simulink model "TractionSystem"  (R2019b)
settings: configuration reference "ConfigSet_TractionSystem_Reference" (kept outside this file)
model workspace (MAT data in the model file):
  Prm_TractionSystem = Simulink.Parameter
  Prm_TractionSystem.Value.DesignMaxTractionTorque = 1091
  Prm_TractionSystem.Value.DesignMaxTractionPower = 210120
  Prm_TractionSystem.Value.DesignTimeToMaxTraction = 1.75
  Prm_TractionSystem.Value.DesignMaxBrakingTorque = 1570
  Prm_TractionSystem.Value.DesignMaxBrakingPower = 430000
  Prm_TractionSystem.Value.BrakeFadeRampDownSpeeds = [0.3 1]
  Prm_TractionSystem.Value.DesignGearingRatio = 6.79
  Prm_TractionSystem.Value.DesignGearingEfficiency = 0.97
  Prm_TractionSystem.Value.DesignWheelDiameter = 0.82
  Prm_TractionSystem.Value.DesignBogieMotorCount = 2
  Prm_TractionSystem.Value.AxleHasMotor = [1 1]
  Prm_TractionSystem.Value.EmergencyBrakeDeactivatesDynamicBrake = 1
  Prm_TractionSystem.Value.WheelSlipProtectionEnable = 1
  Prm_TractionSystem.Value.WheelSlideProtectionEnable = 1
  Prm_TractionSystem.Value.JerkLimit = 0.75
  Prm_TractionSystem.Value.MaxContinuousSlipBeforeTractionCutout = 10
  Prm_TractionSystem.Value.MaxContinuousSlideBeforeBrakeCutout = 10
  Prm_TractionSystem.DataType = 'Bus: BD_TractionSystem_Prm'
  Prm_TractionSystem.Dimensions = [1 1]
  SampleTime = 0.01
undefined symbols (not defined in the file): Audio, BCU, Bogie, BogieNotIsolated, DiscIntNeverNeededParam, Dynamics, EDBrakeStatus, EDBrakingEffortAchieved, EDBrakingEffortPossible, ElectricalSystem, Forward, MaxAxles, Reverse, TCMS, TCUWheelSlideControlActive, TractionContactorStatus, TractionControl, TractionEDPower, Trafo_TCU, VehicleBogieDerailed, VehicleDerailed, WheelAngularVelocity
libraries: simulink x19, LatchesLib x3, TimersLib x2, WheelSlipControl_Lib x2, simulink_extras x2, TractionLib x2
(part 1 of 2)
settings Model: ParameterArgumentNames=Prm_TractionSystem  Creator=cdyer  LastModifiedBy=hinganes
settings ConfigSetRef: SourceName=ConfigSet_TractionSystem_Reference  SourceLocation=Base Workspace

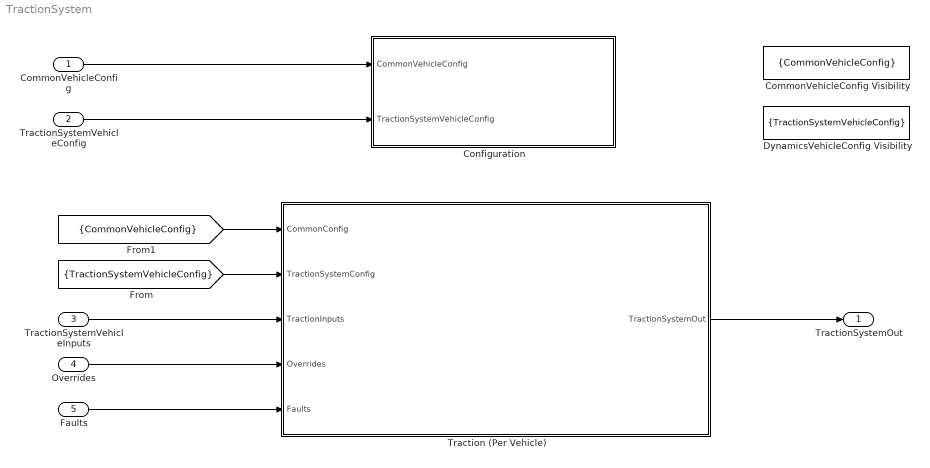
== system TractionSystem ==
  CommonVehicleConfig : Inport  OutDataTypeStr=Bus: BD_CommonTrain_Cfg_Vehicle  PortDimensions=MaxVehicles  BusOutputAsStruct=on
  TractionSystemVehicleConfig : Inport  Port=2  OutDataTypeStr=Bus: BD_TractionSystem_Cfg_Vehicle  BusOutputAsStruct=on
  TractionSystemVehicleInputs : Inport  Port=3  OutDataTypeStr=Bus: BD_TractionSystem_In_Vehicle  BusOutputAsStruct=on
  Overrides : Inport  Port=4  OutDataTypeStr=Bus: BD_TractionSystem_In_Overrides  BusOutputAsStruct=on
  Faults : Inport  Port=5  OutDataTypeStr=Bus: BD_TractionSystem_In_Faults  BusOutputAsStruct=on
  CommonVehicleConfig Visibility : GotoTagVisibility  GotoTag=CommonVehicleConfig
  Configuration : Subsystem
  DynamicsVehicleConfig Visibility : GotoTagVisibility  GotoTag=TractionSystemVehicleConfig
  Traction (Per Vehicle) : Subsystem  TreatAsAtomicUnit=on
  TractionSystemOut : Outport  OutDataTypeStr=Bus: BD_TractionSystem_Out_Vehicle  VectorParamsAs1DForOutWhenUnconnected=off  BusOutputAsStruct=on
  wires:
  Traction (Per Vehicle)/1(TractionSystemOut) -> TractionSystemOut/1
  CommonVehicleConfig/1 -> Configuration/1(CommonVehicleConfig)
  TractionSystemVehicleInputs/1 -> Traction (Per Vehicle)/3(TractionInputs)
  TractionSystemVehicleConfig/1 -> Configuration/2(TractionSystemVehicleConfig)
  [CommonVehicleConfig] -> Traction (Per Vehicle)/1(CommonConfig)
  [TractionSystemVehicleConfig] -> Traction (Per Vehicle)/2(TractionSystemConfig)
  Overrides/1 -> Traction (Per Vehicle)/4(Overrides)
  Faults/1 -> Traction (Per Vehicle)/5(Faults)

== system TractionSystem/Configuration ==
  CommonVehicleConfig : Inport  OutDataTypeStr=Bus: BD_CommonTrain_Cfg_Vehicle  BusOutputAsStruct=on
  TractionSystemVehicleConfig : Inport  Port=2  OutDataTypeStr=Bus: BD_TractionSystem_Cfg_Vehicle  BusOutputAsStruct=on
  ConfigProcessing : Subsystem
  Step : Step  Before=1  After=0  SampleTime=SampleTime
  tag scope: CommonVehicleConfig=scoped, TractionSystemVehicleConfig=scoped
  wires:
  Step/1 -> ConfigProcessing/Enable
  CommonVehicleConfig/1 -> ConfigProcessing/1(In1)
  TractionSystemVehicleConfig/1 -> ConfigProcessing/2(In2)
  ConfigProcessing/1(CommonVehicleConfig) -> [CommonVehicleConfig]
  ConfigProcessing/2(TractionSystemVehicleConfig) -> [TractionSystemVehicleConfig]

== system TractionSystem/Traction (Per Vehicle) ==
  CommonConfig : Inport  Partition=on  PartitionDimension=1  PartitionWidth=1  PartitionOffset=0
  TractionSystemConfig : Inport  Port=2  Partition=on  PartitionDimension=1  PartitionWidth=1  PartitionOffset=0
  TractionInputs : Inport  Port=3  Partition=on  PartitionDimension=1  PartitionWidth=1  PartitionOffset=0
  Overrides : Inport  Port=4  Partition=on  PartitionDimension=1  PartitionWidth=1  PartitionOffset=0
  Faults : Inport  Port=5  Partition=on  PartitionDimension=1  PartitionWidth=1  PartitionOffset=0
  AND : Logic  AllPortsSameDT=off  OutDataTypeStr=boolean
  Bus Selector : BusSelector  OutputSignals=HasMotors
  Bus Selector1 : BusSelector  OutputSignals=Enabled
  ForEachVehicle : ForEach  DisableCoverage=on
  MotorVehicle : Subsystem
  TractionSystemOut : Outport  ConcatenationDimension=1  VectorParamsAs1DForOutWhenUnconnected=off
  wires:
  TractionSystemConfig/1 -> Bus Selector/1
  TractionInputs/1 -> MotorVehicle/2(TractionInputs)
  MotorVehicle/1(TractionSystemOut) -> TractionSystemOut/1
  CommonConfig/1 -> Bus Selector1/1, MotorVehicle/1(CommonConfig)
  Overrides/1 -> MotorVehicle/3(Overrides)
  Faults/1 -> MotorVehicle/4(Faults)
  Bus Selector/1 -> AND/1  "<HasMotors>"
  Bus Selector1/1 -> AND/2  "<Enabled>"
  AND/1 -> MotorVehicle/Enable

== system TractionSystem/Configuration/ConfigProcessing ==
  In1 : Inport
  In2 : Inport  Port=2
  Enable : EnablePort
  ConfigCheck : Subsystem
  CommonVehicleConfig : Outport  VectorParamsAs1DForOutWhenUnconnected=off  BusOutputAsStruct=on
  TractionSystemVehicleConfig : Outport  Port=2  VectorParamsAs1DForOutWhenUnconnected=off  BusOutputAsStruct=on
  wires:
  In1/1 -> ConfigCheck/1(In1)
  In2/1 -> ConfigCheck/2(In2)
  ConfigCheck/1(CommonVehicleConfig) -> CommonVehicleConfig/1
  ConfigCheck/2(TractionSystemVehicleConfig) -> TractionSystemVehicleConfig/1

== system TractionSystem/Traction (Per Vehicle)/MotorVehicle ==
  CommonConfig : Inport
  TractionInputs : Inport  Port=2
  Overrides : Inport  Port=3
  Faults : Inport  Port=4
  MotorVehicleEnable : EnablePort
  OutputAdapter : Subsystem
  Unit Delay : UnitDelay  SampleTime=-1  HasFrameUpgradeWarning=on
  VehicleTractionControlUnit : Subsystem
  VehicleTractionConvertersSystem : Subsystem
  TractionSystemOut : Outport  VectorParamsAs1DForOutWhenUnconnected=off
  wires:
  Faults/1 -> VehicleTractionConvertersSystem/5(Faults), VehicleTractionControlUnit/2(Faults)
  Overrides/1 -> VehicleTractionControlUnit/3(Overrides), VehicleTractionConvertersSystem/4(Overrides)
  CommonConfig/1 -> VehicleTractionConvertersSystem/3(CommonConfig)
  VehicleTractionControlUnit/2(TractionConverterControl) -> VehicleTractionConvertersSystem/1(TractionConverterControlIn)
  VehicleTractionConvertersSystem/2(BogieOutputs) -> Unit Delay/1
  Unit Delay/1 -> VehicleTractionControlUnit/4(TractionConvertersFB)
  VehicleTractionConvertersSystem/1(VehicleTractiveBrakingEffortPerAxle) -> OutputAdapter/3(VehicleTractiveBrakingEffortPerAxle)
  OutputAdapter/1(TractionSystemOut) -> TractionSystemOut/1
  TractionInputs/1 -> VehicleTractionConvertersSystem/2(TractionInputs), VehicleTractionControlUnit/1(TractionInputs), OutputAdapter/1(TractionInputs)
  VehicleTractionControlUnit/1(TractionControlUnitOut) -> OutputAdapter/2(TractionControlUnitOut)

== system TractionSystem/Configuration/ConfigProcessing/ConfigCheck ==
  In1 : Inport  Partition=on  PartitionDimension=1  PartitionWidth=1  PartitionOffset=0
  In2 : Inport  Port=2  Partition=on  PartitionDimension=1  PartitionWidth=1  PartitionOffset=0
  Bus Creator1 : BusCreator  Inputs=1  OutDataTypeStr=Bus: BD_TractionSystem_Cfg_Vehicle  NonVirtualBus=on
      settings: InheritFromInputs=off
  Bus Creator2 : BusCreator  Inputs=15  OutDataTypeStr=Bus: BD_CommonTrain_Cfg_Vehicle  NonVirtualBus=on
      settings: InheritFromInputs=off
  Bus Selector1 : BusSelector  OutputSignals=HasMotors
  Bus Selector3 : BusSelector  OutputSignals=Enabled,VehicleID,Type,Class,Orientation,Length,Height,Width,TareMass,GrossMass,LoadingMass,NumberOfAxles,NumberOfDrivenAxles,NumberOfBrakedAxles,WheelDiameter
  Data Type Conversion : DataTypeConversion
  Default Gearing Ratio : Subsystem
  Default Gross1 : Subsystem
  Default Height1 : Subsystem
  Default Length1 : Subsystem
  Default NumberOfAxles3 : Subsystem
  Default NumberOfAxles4 : Subsystem
  Default NumberOfAxles5 : Subsystem
  Default Tare1 : Subsystem
  Default WheelDiameter : Subsystem
  Default Width1 : Subsystem
  For Each : ForEach  DisableCoverage=on
  CommonVehicleConfig : Outport  ConcatenationDimension=1  VectorParamsAs1DForOutWhenUnconnected=off
  TractionSystemVehicleConfig : Outport  Port=2  ConcatenationDimension=1  VectorParamsAs1DForOutWhenUnconnected=off
  wires:
  In2/1 -> Bus Selector1/1
  Bus Selector1/1 -> Default Gearing Ratio/1(In1)  "<HasMotors>"
  Data Type Conversion/1 -> Bus Creator1/1  "HasMotors"
  Bus Creator1/1 -> TractionSystemVehicleConfig/1
  In1/1 -> Bus Selector3/1
  Bus Selector3/3 -> Bus Creator2/3  "<Type>"
  Bus Selector3/4 -> Bus Creator2/4  "<Class>"
  Bus Selector3/5 -> Bus Creator2/5  "<Orientation>"
  Bus Selector3/6 -> Default Length1/1(In1)  "<Length>"
  Bus Selector3/7 -> Default Height1/1(In1)  "<Height>"
  Bus Selector3/8 -> Default Width1/1(In1)  "<Width>"
  Bus Selector3/9 -> Default Tare1/1(In1)  "<TareMass>"
  Bus Selector3/10 -> Default Gross1/1(In1)  "<GrossMass>"
  Bus Selector3/11 -> Bus Creator2/11  "<LoadingMass>"
  Default Length1/1(Out1) -> Bus Creator2/6  "Length"
  Bus Creator2/1 -> CommonVehicleConfig/1
  Default Height1/1(Out1) -> Bus Creator2/7  "Height"
  Default Width1/1(Out1) -> Bus Creator2/8  "Width"
  Default Tare1/1(Out1) -> Bus Creator2/9  "TareMass"
  Default Gross1/1(Out1) -> Bus Creator2/10  "GrossMass"
  Bus Selector3/12 -> Default NumberOfAxles3/1(In)  "<NumberOfAxles>"
  Default NumberOfAxles3/1(Out) -> Bus Creator2/12  "NumberOfAxles"
  Bus Selector3/13 -> Default NumberOfAxles4/1(In)  "<NumberOfDrivenAxles>"
  Bus Selector3/14 -> Default NumberOfAxles5/1(In)  "<NumberOfBrakedAxles>"
  Default NumberOfAxles5/1(Out) -> Bus Creator2/14  "NumberOfBrakedAxles"
  Default NumberOfAxles4/1(Out) -> Bus Creator2/13  "NumberOfDrivenAxles"
  Bus Selector3/15 -> Default WheelDiameter/1(In)  "<WheelDiameter>"
  Bus Selector3/1 -> Bus Creator2/1  "<Enabled>"
  Default WheelDiameter/1(Out) -> Bus Creator2/15  "WheelDiameter"
  Bus Selector3/2 -> Bus Creator2/2  "<VehicleID>"
  Default Gearing Ratio/1(Out1) -> Data Type Conversion/1  "HasMotors"

== system TractionSystem/Traction (Per Vehicle)/MotorVehicle/OutputAdapter ==
  TractionInputs : Inport
  TractionControlUnitOut : Inport  Port=2
  VehicleTractiveBrakingEffortPerAxle : Inport  Port=3
  AudioOutputsRepack : Subsystem
  Bus Assignment : BusAssignment  AssignedSignals=TractionControl,Dynamics,Audio
  Constant1 : Constant  Value=0  OutDataTypeStr=Bus: BD_TractionSystem_Out_Vehicle
  DynamicsOutputsRepack : Subsystem
  TractionSystemOut : Outport  VectorParamsAs1DForOutWhenUnconnected=off
  wires:
  Bus Assignment/1 -> TractionSystemOut/1
  Constant1/1 -> Bus Assignment/1
  VehicleTractiveBrakingEffortPerAxle/1 -> AudioOutputsRepack/1(In1), DynamicsOutputsRepack/1(VehicleTractiveBrakingEffortPerAxle)
  DynamicsOutputsRepack/1(DynamicsTractionBrakingForce) -> Bus Assignment/3
  TractionInputs/1 -> AudioOutputsRepack/2(TractionInputs)
  AudioOutputsRepack/1(Out1) -> Bus Assignment/4
  TractionControlUnitOut/1 -> Bus Assignment/2

== system TractionSystem/Traction (Per Vehicle)/MotorVehicle/VehicleTractionControlUnit ==
  TractionInputs : Inport
  Faults : Inport  Port=2
  Overrides : Inport  Port=3
  TractionConvertersFB : Inport  Port=4
  Bus Selector : BusSelector  OutputSignals=ElectricalSystem,Dynamics,TCMS
  Bus Selector1 : BusSelector  OutputSignals=ForwardTW,ReverseTW,TractionActiveTW,NoEmergencyBrakeActiveTW,VCBState,ContactorsFailure,Bogie
  Bus Selector2 : BusSelector  OutputSignals=Velocity,Bogie
  Bus Selector3 : BusSelector  OutputSignals=TCMSTractionCmd,TCMSEDBrakingCmd,Bogie
  Bus Selector4 : BusSelector  OutputSignals=Bogie
  OutputAdapter : Subsystem
  Subsystem : Subsystem
  Sum of Elements : Sum  Inputs=+
  Terminator : Terminator
  TractionControl (Per Bogie) : Subsystem
  TractionConverterCircuits : Subsystem
  TractionControlUnitOut : Outport  VectorParamsAs1DForOutWhenUnconnected=off
  TractionConverterControl : Outport  Port=2  VectorParamsAs1DForOutWhenUnconnected=off
  wires:
  TractionInputs/1 -> Bus Selector/1
  Faults/1 -> TractionControl (Per Bogie)/15(Faults), OutputAdapter/6(Faults), Bus Selector4/1, TractionConverterCircuits/3(Faults)
  Overrides/1 -> TractionControl (Per Bogie)/13(Overrides)
  TractionConvertersFB/1 -> Subsystem/1(In1), TractionControl (Per Bogie)/14(TractionConvertersFB)
  TractionControl (Per Bogie)/2(TCUtoElectricalOutputs) -> OutputAdapter/1(TCUtoElectricalOut)
  TractionControl (Per Bogie)/1(TractionConverterControl) -> TractionConverterControl/1
  Bus Selector/1 -> Bus Selector1/1  "<ElectricalSystem>"
  Bus Selector/2 -> Bus Selector2/1  "<Dynamics>"
  Bus Selector/3 -> Bus Selector3/1  "<TCMS>"
  Bus Selector1/1 -> TractionControl (Per Bogie)/1(ForwardTW)  "<ForwardTW>"
  Bus Selector1/2 -> TractionControl (Per Bogie)/2(ReverseTW)  "<ReverseTW>"
  Bus Selector1/3 -> TractionControl (Per Bogie)/3(TractionActive)  "<TractionActiveTW>"
  Bus Selector1/4 -> TractionControl (Per Bogie)/4(NoEmergencyBrakeActive)  "<NoEmergencyBrakeActiveTW>"
  Bus Selector1/7 -> TractionControl (Per Bogie)/6(BogieElectrical)  "<Bogie>"
  Bus Selector2/1 -> TractionControl (Per Bogie)/7(Velocity)  "<Velocity>"
  Bus Selector2/2 -> TractionControl (Per Bogie)/8(BogieDynamics)  "<Bogie>"
  Bus Selector3/1 -> TractionControl (Per Bogie)/9(TCMSTractionCmd)  "<TCMSTractionCmd>"
  Bus Selector3/2 -> TractionControl (Per Bogie)/10(TCMSEDBrakingCmd)  "<TCMSEDBrakingCmd>"
  TractionControl (Per Bogie)/4(TCUToBCUOutputs) -> OutputAdapter/3(TCUtoBCUOut)
  Bus Selector3/3 -> TractionControl (Per Bogie)/11(TCMSBogie)  "<Bogie>"
  TractionControl (Per Bogie)/3(TCUtoTCMSOutputs) -> OutputAdapter/2(TCUtoTCMSOut)
  OutputAdapter/1(TractionControlUnitOut) -> TractionControlUnitOut/1
  Bus Selector4/1 -> TractionControl (Per Bogie)/12(BogieFaults)  "<Bogie>"
  Bus Selector1/5 -> TractionConverterCircuits/1(VCB State)  "<VCBState>"
  TractionConverterCircuits/1(TMPower) -> [ContactorStatus], TractionControl (Per Bogie)/5(TMPower)
  TractionConverterCircuits/2(Trafo_TCU) -> OutputAdapter/5(Trafo_TCU)
  Sum of Elements/1 -> Terminator/1  "VehicleTractivePower"
  Subsystem/1(<BogieTractivePower>) -> Sum of Elements/1
  Bus Selector1/6 -> TractionConverterCircuits/2(ContactorFault)  "<ContactorsFailure>"
  [ContactorStatus] -> OutputAdapter/4(ContactorStatus)

== system TractionSystem/Traction (Per Vehicle)/MotorVehicle/VehicleTractionConvertersSystem ==
  TractionConverterControlIn : Inport
  Bus Element In : Inport  Port=2  PortName=TractionInputs  Element=Dynamics
  In Bus Element : Inport  Port=2  PortName=TractionInputs  Element=ElectricalSystem
  In Bus Element1 : Inport  Port=2  PortName=TractionInputs  Element=TCMS
  CommonConfig : Inport  Port=3
  Overrides : Inport  Port=4
  Faults : Inport  Port=5
  BogieTractionConverterSystem (Per Bogie) : Subsystem
  Bus Selector1 : BusSelector  OutputSignals=Bogie
  Bus Selector2 : BusSelector  OutputSignals=Orientation
  Bus Selector5 : BusSelector  OutputSignals=TractionForceVariation,DynamicBrakeForceVariation
  Terminator1 : Terminator
  VehicleTractiveBrakingEffortPerAxle : Outport  VectorParamsAs1DForOutWhenUnconnected=off
  BogieOutputs : Outport  Port=2  VectorParamsAs1DForOutWhenUnconnected=off
  wires:
  TractionConverterControlIn/1 -> BogieTractionConverterSystem (Per Bogie)/1(BogieTractionConverterControlIn)
  Bus Element In/1 -> Bus Selector1/1
  Overrides/1 -> Bus Selector5/1
  CommonConfig/1 -> Bus Selector2/1
  Bus Selector5/1 -> BogieTractionConverterSystem (Per Bogie)/4(TractionEffortVariationOverride)  "<TractionForceVariation>"
  Bus Selector5/2 -> BogieTractionConverterSystem (Per Bogie)/5(BrakingEffortVariationOverride)  "<DynamicBrakeForceVariation>"
  Bus Selector1/1 -> BogieTractionConverterSystem (Per Bogie)/3(BogieDynamics)  "<Bogie>"
  Bus Selector2/1 -> BogieTractionConverterSystem (Per Bogie)/6(Orientation)  "<Orientation>"
  BogieTractionConverterSystem (Per Bogie)/1(BogieForcesPerAxle) -> VehicleTractiveBrakingEffortPerAxle/1
  Faults/1 -> Terminator1/1
  BogieTractionConverterSystem (Per Bogie)/2(BogieOutputs) -> BogieOutputs/1
  In Bus Element/1 -> BogieTractionConverterSystem (Per Bogie)/2(MotorIn)
  In Bus Element1/1 -> BogieTractionConverterSystem (Per Bogie)/7(TCMS)

== system TractionSystem/Configuration/ConfigProcessing/ConfigCheck/Default Gearing Ratio ==
  In1 : Inport
  Default : Constant  Value=0
  Min Value : simulink/Logic and Bit Operations/Compare To Constant  relop=>  const=0  OutDataTypeStr=boolean
  Switch : Switch  Criteria=u2 > Threshold
  Out1 : Outport  VectorParamsAs1DForOutWhenUnconnected=off
  wires:
  In1/1 -> Min Value/1, Switch/1
  Min Value/1 -> Switch/2
  Default/1 -> Switch/3
  Switch/1 -> Out1/1

== system TractionSystem/Configuration/ConfigProcessing/ConfigCheck/Default Gross1 ==
  In1 : Inport
  Default : Constant  Value=16000
  Min Value : simulink/Logic and Bit Operations/Compare To Constant  relop=>  const=16000  OutDataTypeStr=boolean
  Switch : Switch  Criteria=u2 > Threshold
  Out1 : Outport  VectorParamsAs1DForOutWhenUnconnected=off
  wires:
  In1/1 -> Min Value/1, Switch/1
  Min Value/1 -> Switch/2
  Default/1 -> Switch/3
  Switch/1 -> Out1/1

== system TractionSystem/Configuration/ConfigProcessing/ConfigCheck/Default Height1 ==
  In1 : Inport
  Default : Constant  Value=3
  Min Value : simulink/Logic and Bit Operations/Compare To Constant  relop=>  const=0  OutDataTypeStr=boolean
  Switch : Switch  Criteria=u2 > Threshold
  Out1 : Outport  VectorParamsAs1DForOutWhenUnconnected=off
  wires:
  In1/1 -> Min Value/1, Switch/1
  Min Value/1 -> Switch/2
  Default/1 -> Switch/3
  Switch/1 -> Out1/1

== system TractionSystem/Configuration/ConfigProcessing/ConfigCheck/Default Length1 ==
  In1 : Inport
  Default : Constant  Value=20
  Min Value : simulink/Logic and Bit Operations/Compare To Constant  relop=>  const=0  OutDataTypeStr=boolean
  Switch : Switch  Criteria=u2 > Threshold
  Out1 : Outport  VectorParamsAs1DForOutWhenUnconnected=off
  wires:
  In1/1 -> Min Value/1, Switch/1
  Min Value/1 -> Switch/2
  Default/1 -> Switch/3
  Switch/1 -> Out1/1

== system TractionSystem/Configuration/ConfigProcessing/ConfigCheck/Default NumberOfAxles3 ==
  In : Inport
  Default : Constant  Value=6
  Min Value : simulink/Logic and Bit Operations/Compare To Constant  relop=>=  const=1  OutDataTypeStr=boolean
  Switch : Switch  Criteria=u2 > Threshold
  Out : Outport  VectorParamsAs1DForOutWhenUnconnected=off
  wires:
  Switch/1 -> Out/1
  Default/1 -> Switch/3
  Min Value/1 -> Switch/2
  In/1 -> Switch/1, Min Value/1

== system TractionSystem/Configuration/ConfigProcessing/ConfigCheck/Default NumberOfAxles4 ==
  In : Inport
  Default : Constant  Value=2
  Min Value : simulink/Logic and Bit Operations/Compare To Constant  relop=>=  const=1  OutDataTypeStr=boolean
  Switch : Switch  Criteria=u2 > Threshold
  Out : Outport  VectorParamsAs1DForOutWhenUnconnected=off
  wires:
  In/1 -> Min Value/1, Switch/1
  Min Value/1 -> Switch/2
  Default/1 -> Switch/3
  Switch/1 -> Out/1

== system TractionSystem/Configuration/ConfigProcessing/ConfigCheck/Default NumberOfAxles5 ==
  In : Inport
  Default : Constant  Value=2
  Min Value : simulink/Logic and Bit Operations/Compare To Constant  relop=>=  const=1  OutDataTypeStr=boolean
  Switch : Switch  Criteria=u2 > Threshold
  Out : Outport  VectorParamsAs1DForOutWhenUnconnected=off
  wires:
  Switch/1 -> Out/1
  Default/1 -> Switch/3
  Min Value/1 -> Switch/2
  In/1 -> Switch/1, Min Value/1

== system TractionSystem/Configuration/ConfigProcessing/ConfigCheck/Default Tare1 ==
  In1 : Inport
  Default : Constant  Value=16000
  Min Value : simulink/Logic and Bit Operations/Compare To Constant  relop=>  const=16000  OutDataTypeStr=boolean
  Switch : Switch  Criteria=u2 > Threshold
  Out1 : Outport  VectorParamsAs1DForOutWhenUnconnected=off
  wires:
  In1/1 -> Min Value/1, Switch/1
  Min Value/1 -> Switch/2
  Default/1 -> Switch/3
  Switch/1 -> Out1/1

== system TractionSystem/Configuration/ConfigProcessing/ConfigCheck/Default WheelDiameter ==
  In : Inport
  Default : Constant  Value=0.580
  Min Value : simulink/Logic and Bit Operations/Compare To Constant  relop=>  const=0  OutDataTypeStr=boolean
  Switch : Switch  Criteria=u2 > Threshold
  Out : Outport  VectorParamsAs1DForOutWhenUnconnected=off
  wires:
  In/1 -> Min Value/1, Switch/1
  Min Value/1 -> Switch/2
  Default/1 -> Switch/3
  Switch/1 -> Out/1

== system TractionSystem/Configuration/ConfigProcessing/ConfigCheck/Default Width1 ==
  In1 : Inport
  Default : Constant  Value=3
  Min Value : simulink/Logic and Bit Operations/Compare To Constant  relop=>  const=0  OutDataTypeStr=boolean
  Switch : Switch  Criteria=u2 > Threshold
  Out1 : Outport  VectorParamsAs1DForOutWhenUnconnected=off
  wires:
  In1/1 -> Min Value/1, Switch/1
  Min Value/1 -> Switch/2
  Default/1 -> Switch/3
  Switch/1 -> Out1/1

== system TractionSystem/Traction (Per Vehicle)/MotorVehicle/OutputAdapter/AudioOutputsRepack ==
  In1 : Inport
  TractionInputs : Inport  Port=2
  Bus Assignment1 : BusAssignment  AssignedSignals=TractionEDPower,WheelAngularVelocity
  Bus Selector : BusSelector  OutputSignals=Dynamics.Bogie
  Constant : Constant  Value=Prm_TractionSystem.DesignWheelDiameter
  Constant2 : Constant  Value=0  OutDataTypeStr=Bus: BD_TractionSystem_Out_Vehicle_Audio
  ForEachBogie : Subsystem  TreatAsAtomicUnit=on
  Gain : Gain  Gain=0.5
  IfWheelSlipping : MinMax  Function=max
  Product : Product  Inputs=*/
  Sum of Elements : Sum  Inputs=+
  Out1 : Outport
  wires:
  Gain/1 -> Product/2
  IfWheelSlipping/1 -> Product/1
  ForEachBogie/1(BogieTractionBrakingPower) -> Sum of Elements/1
  TractionInputs/1 -> Bus Selector/1
  ForEachBogie/2(BogieWheelSpeed) -> IfWheelSlipping/1
  Bus Selector/1 -> ForEachBogie/2(BogieDynamics)  "<Bogie>"
  Constant2/1 -> Bus Assignment1/1
  Product/1 -> Bus Assignment1/3  "WheelAngularSpeed"
  Sum of Elements/1 -> Bus Assignment1/2
  Constant/1 -> Gain/1
  Bus Assignment1/1 -> Out1/1
  In1/1 -> ForEachBogie/1(BogieTraction)

== system TractionSystem/Traction (Per Vehicle)/MotorVehicle/OutputAdapter/DynamicsOutputsRepack ==
  VehicleTractiveBrakingEffortPerAxle : Inport
  Assignment : Assignment  DiagnosticForDimensions=Warning  IndexOptions=Starting index (dialog)  Indices=1  OutputSizes=1
  Assignment1 : Assignment  DiagnosticForDimensions=Warning  IndexOptions=Starting index (dialog)  Indices=1  OutputSizes=1
  Assignment2 : Assignment  DiagnosticForDimensions=Warning  IndexOptions=Starting index (dialog)  Indices=1  OutputSizes=1
  Bus Creator : BusCreator  Inputs=3  OutDataTypeStr=Bus: BD_TractionSystem_Out_Vehicle_Dynamics  NonVirtualBus=on
  Constant : Constant  Value=zeros(1,MaxAxles)
  For Each Subsystem : Subsystem  TreatAsAtomicUnit=on
  DynamicsTractionBrakingForce : Outport
  wires:
  Constant/1 -> Assignment2/1, Assignment1/1, Assignment/1
  Bus Creator/1 -> DynamicsTractionBrakingForce/1
  Assignment/1 -> Bus Creator/1  "TractionBrakingForce"
  VehicleTractiveBrakingEffortPerAxle/1 -> For Each Subsystem/1(In1)
  For Each Subsystem/1(TractionBrakingForce) -> Assignment/2
  Assignment1/1 -> Bus Creator/2  "TractionForce"
  Assignment2/1 -> Bus Creator/3  "BrakingForce"
  For Each Subsystem/2(TractionForce) -> Assignment1/2
  For Each Subsystem/3(BrakingForce) -> Assignment2/2

== system TractionSystem/Traction (Per Vehicle)/MotorVehicle/VehicleTractionControlUnit/OutputAdapter ==
  TCUtoElectricalOut : Inport
  TCUtoTCMSOut : Inport  Port=2
  TCUtoBCUOut : Inport  Port=3
  ContactorStatus : Inport  Port=4
  In Bus Element : Inport  Port=5  PortName=Trafo_TCU
  Faults : Inport  Port=6
  BCUOutputsRepack : Subsystem
  Bus Assignment : BusAssignment  AssignedSignals=ElectricalSystem,TCMS,BCU
  Constant1 : Constant  Value=0  OutDataTypeStr=Bus: BD_TractionSystem_Out_Vehicle_TCU
  ElectricalOutputsRepack : Subsystem
  TCMSOutputsRepack : Subsystem
  TractionControlUnitOut : Outport  VectorParamsAs1DForOutWhenUnconnected=off
  wires:
  Bus Assignment/1 -> TractionControlUnitOut/1
  Constant1/1 -> Bus Assignment/1
  TCUtoElectricalOut/1 -> ElectricalOutputsRepack/2(In1)
  ElectricalOutputsRepack/1(ToElectrical) -> Bus Assignment/2
  TCUtoTCMSOut/1 -> TCMSOutputsRepack/1(In1)
  TCMSOutputsRepack/1(ToTCMS) -> Bus Assignment/3
  BCUOutputsRepack/1(ToBCU) -> Bus Assignment/4
  TCUtoBCUOut/1 -> BCUOutputsRepack/1(In1)
  In Bus Element/1 -> TCMSOutputsRepack/2(In2)
  ContactorStatus/1 -> ElectricalOutputsRepack/1(In2)
  Faults/1 -> TCMSOutputsRepack/3(In3)

== system TractionSystem/Traction (Per Vehicle)/MotorVehicle/VehicleTractionControlUnit/Subsystem ==
  In1 : Inport  Partition=on  PartitionDimension=1  PartitionWidth=1  PartitionOffset=0
  Bus Selector5 : BusSelector  OutputSignals=BogieTractivePower
  ForEachBogie : ForEach  DisableCoverage=on
  <BogieTractivePower> : Outport  ConcatenationDimension=1
  wires:
  Bus Selector5/1 -> <BogieTractivePower>/1  "<BogieTractivePower>"
  In1/1 -> Bus Selector5/1

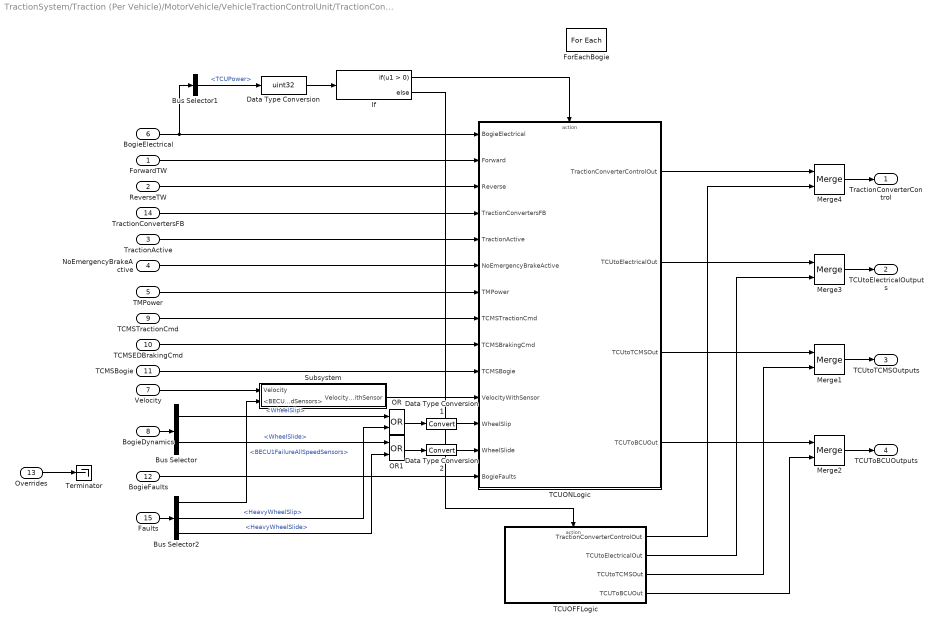
== system TractionSystem/Traction (Per Vehicle)/MotorVehicle/VehicleTractionControlUnit/TractionControl (Per Bogie) ==
  ForwardTW : Inport
  ReverseTW : Inport  Port=2
  TractionActive : Inport  Port=3
  NoEmergencyBrakeActive : Inport  Port=4
  TMPower : Inport  Port=5
  BogieElectrical : Inport  Port=6  Partition=on  PartitionDimension=1  PartitionWidth=1  PartitionOffset=0
  Velocity : Inport  Port=7
  BogieDynamics : Inport  Port=8  Partition=on  PartitionDimension=1  PartitionWidth=1  PartitionOffset=0
  TCMSTractionCmd : Inport  Port=9
  TCMSEDBrakingCmd : Inport  Port=10
  TCMSBogie : Inport  Port=11  Partition=on  PartitionDimension=1  PartitionWidth=1  PartitionOffset=0
  BogieFaults : Inport  Port=12  Partition=on  PartitionDimension=1  PartitionWidth=1  PartitionOffset=0
  Overrides : Inport  Port=13
  TractionConvertersFB : Inport  Port=14  Partition=on  PartitionDimension=1  PartitionWidth=1  PartitionOffset=0
  Faults : Inport  Port=15
  Bus Selector : BusSelector  OutputSignals=WheelSlip,WheelSlide
  Bus Selector1 : BusSelector  OutputSignals=TCUPower
  Bus Selector2 : BusSelector  OutputSignals=BECU1FailureAllSpeedSensors,HeavyWheelSlip,HeavyWheelSlide
  Data Type Conversion : DataTypeConversion  OutDataTypeStr=uint32
  Data Type Conversion1 : DataTypeConversion
  Data Type Conversion2 : DataTypeConversion
  ForEachBogie : ForEach  DisableCoverage=on
  If : If
  Merge{1..4} (4 alike) : Merge
  OR : Logic  Operator=OR  AllPortsSameDT=off  OutDataTypeStr=boolean
  OR1 : Logic  Operator=OR  AllPortsSameDT=off  OutDataTypeStr=boolean
  Subsystem : Subsystem
  TCUOFFLogic : Subsystem  TreatAsAtomicUnit=on
  TCUONLogic : Subsystem
  Terminator : Terminator
  TractionConverterControl : Outport  ConcatenationDimension=1  VectorParamsAs1DForOutWhenUnconnected=off
  TCUtoElectricalOutputs : Outport  Port=2  ConcatenationDimension=1  VectorParamsAs1DForOutWhenUnconnected=off
  TCUtoTCMSOutputs : Outport  Port=3  ConcatenationDimension=1
  TCUToBCUOutputs : Outport  Port=4  ConcatenationDimension=1
  wires:
  TractionConvertersFB/1 -> TCUONLogic/4(TractionConvertersFB)
  ForwardTW/1 -> TCUONLogic/2(Forward)
  ReverseTW/1 -> TCUONLogic/3(Reverse)
  BogieElectrical/1 -> Bus Selector1/1, TCUONLogic/1(BogieElectrical)
  TractionActive/1 -> TCUONLogic/5(TractionActive)
  NoEmergencyBrakeActive/1 -> TCUONLogic/6(NoEmergencyBrakeActive)
  Overrides/1 -> Terminator/1
  BogieFaults/1 -> TCUONLogic/14(BogieFaults)
  TCMSTractionCmd/1 -> TCUONLogic/8(TCMSTractionCmd)
  TCMSEDBrakingCmd/1 -> TCUONLogic/9(TCMSBrakingCmd)
  BogieDynamics/1 -> Bus Selector/1
  Bus Selector/1 -> OR/1  "<WheelSlip>"
  Bus Selector/2 -> OR1/1  "<WheelSlide>"
  Merge2/1 -> TCUToBCUOutputs/1
  TCMSBogie/1 -> TCUONLogic/10(TCMSBogie)
  Bus Selector1/1 -> Data Type Conversion/1  "<TCUPower>"
  If/1 -> TCUONLogic/Action
  TCUONLogic/4(TCUToBCUOut) -> Merge2/1
  Merge1/1 -> TCUtoTCMSOutputs/1
  Merge3/1 -> TCUtoElectricalOutputs/1
  Merge4/1 -> TractionConverterControl/1
  TCUONLogic/3(TCUtoTCMSOut) -> Merge1/1
  TCUONLogic/1(TractionConverterControlOut) -> Merge4/1
  TCUONLogic/2(TCUtoElectricalOut) -> Merge3/1
  TCUOFFLogic/1(TractionConverterControlOut) -> Merge4/2
  TCUOFFLogic/2(TCUtoElectricalOut) -> Merge3/2
  TCUOFFLogic/3(TCUtoTCMSOut) -> Merge1/2
  TCUOFFLogic/4(TCUToBCUOut) -> Merge2/2
  If/2 -> TCUOFFLogic/Action
  Data Type Conversion/1 -> If/1
  TMPower/1 -> TCUONLogic/7(TMPower)
  Faults/1 -> Bus Selector2/1
  Bus Selector2/2 -> OR/2  "<HeavyWheelSlip>"
  OR/1 -> Data Type Conversion1/1
  Data Type Conversion1/1 -> TCUONLogic/12(WheelSlip)
  OR1/1 -> Data Type Conversion2/1
  Data Type Conversion2/1 -> TCUONLogic/13(WheelSlide)
  Bus Selector2/3 -> OR1/2  "<HeavyWheelSlide>"
  Velocity/1 -> Subsystem/1(Velocity)
  Bus Selector2/1 -> Subsystem/2(<BECU1FailureAllSpeedSensors>)  "<BECU1FailureAllSpeedSensors>"
  Subsystem/1(VelocityWithSensor) -> TCUONLogic/11(VelocityWithSensor)

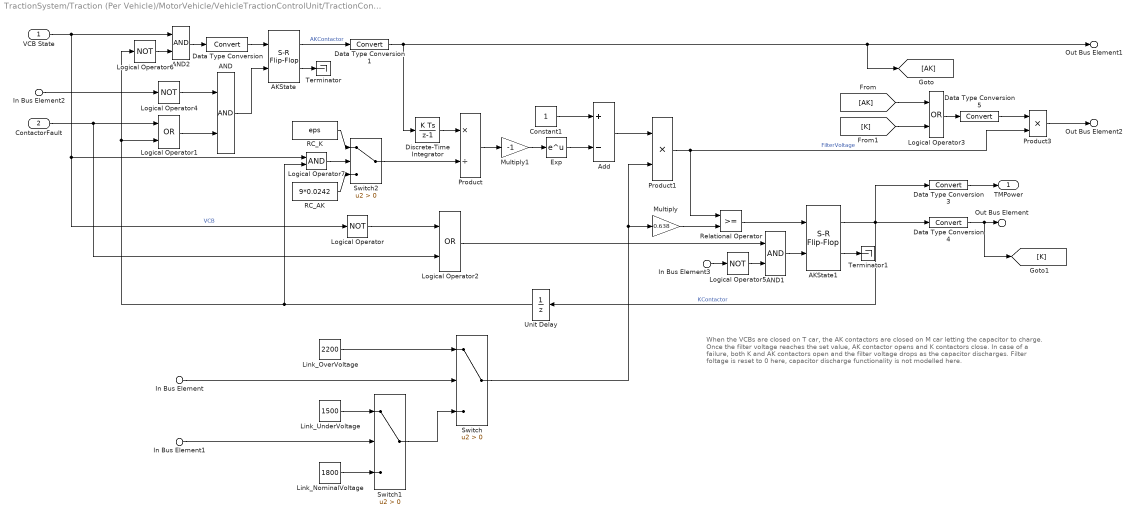
== system TractionSystem/Traction (Per Vehicle)/MotorVehicle/VehicleTractionControlUnit/TractionConverterCircuits ==
  note: When the VCBs are closed on T car, the AK contactors are closed on M car letting the capacitor to charge.
      | Once the filter voltage reaches the set value, AK contactor opens and K contactors close.
      | In case of a failure, both K and AK contactors open and the filter voltage drops as the capacitor discharges.
      | Filter foltage is reset to 0 here, capacitor discharge functionality is not modelled here.
  VCB State : Inport
  ContactorFault : Inport  Port=2
  In Bus Element : Inport  Port=3  PortName=Faults  Element=DCLinkOverVoltageLevel1
  In Bus Element1 : Inport  Port=3  PortName=Faults  Element=DCLinkLowVoltageLevel1
  In Bus Element2 : Inport  Port=3  PortName=Faults  Element=CIAKOpenFailure
  In Bus Element3 : Inport  Port=3  PortName=Faults  Element=CIKOpenFailure
  AKState : simulink_extras/Flip Flops/S-R Flip-Flop  initial_condition=0
  AKState1 : simulink_extras/Flip Flops/S-R Flip-Flop  initial_condition=0
  AND : Logic  AllPortsSameDT=off  OutDataTypeStr=boolean
  AND1 : Logic  AllPortsSameDT=off  OutDataTypeStr=boolean
  AND2 : Logic  AllPortsSameDT=off  OutDataTypeStr=boolean
  Add : Sum  Inputs=+-
  Constant1 : Constant
  Data Type Conversion{,1,3..5} (5 alike) : DataTypeConversion
  Discrete-Time Integrator : DiscreteIntegrator  SampleTime=0.01  ICPrevOutput=DiscIntNeverNeededParam  ICPrevScaledInput=DiscIntNeverNeededParam
  Exp : Math  SignedPower=off  SaturateOnIntegerOverflow=on
  Link_NominalVoltage : Constant  Value=1800
  Link_OverVoltage : Constant  Value=2200
  Link_UnderVoltage : Constant  Value=1500
  Logical Operator{,4..6} (4 alike) : Logic  Operator=NOT  AllPortsSameDT=off  OutDataTypeStr=boolean
  Logical Operator1 : Logic  Operator=OR  AllPortsSameDT=off  OutDataTypeStr=boolean
  Logical Operator2 : Logic  Operator=OR  AllPortsSameDT=off  OutDataTypeStr=boolean
  Logical Operator3 : Logic  Operator=OR  AllPortsSameDT=off  OutDataTypeStr=boolean
  Logical Operator7 : Logic  AllPortsSameDT=off  OutDataTypeStr=boolean
  Multiply : Gain  Gain=0.638
  Multiply1 : Gain  Gain=-1
  Product : Product  Inputs=*/
  Product1 : Product  Inputs=**
  Product3 : Product  Inputs=**
  RC_AK : Constant  Value=9*0.0242
  RC_K : Constant  Value=eps
  Relational Operator : RelationalOperator  OutDataTypeStr=boolean  RndMeth=Simplest
  Switch : Switch  Criteria=u2 > Threshold
  Switch1 : Switch  Criteria=u2 > Threshold
  Switch2 : Switch  Criteria=u2 > Threshold
  Terminator : Terminator
  Terminator1 : Terminator
  Unit Delay : UnitDelay  SampleTime=-1  HasFrameUpgradeWarning=on
  TMPower : Outport
  Out Bus Element : Outport  Port=2  PortName=Trafo_TCU  Element=TCU_KStatus
  Out Bus Element1 : Outport  Port=2  PortName=Trafo_TCU  Element=TCU_AKStatus
  Out Bus Element2 : Outport  Port=2  PortName=Trafo_TCU  Element=FilterVoltage
  wires:
  VCB State/1 -> Logical Operator7/1, Logical Operator/1, AND2/1  "VCB"
  AKState/1 -> Data Type Conversion1/1  "AKContactor"
  Discrete-Time Integrator/1 -> Product/1
  Product/1 -> Multiply1/1
  Exp/1 -> Add/2
  Constant1/1 -> Add/1
  Add/1 -> Product1/1
  Switch/1 -> Product1/2, Multiply/1
  Product1/1 -> Product3/2, Relational Operator/1  "FilterVoltage"
  AKState/2 -> Terminator/1
  Data Type Conversion1/1 -> Discrete-Time Integrator/1, [AK], Out Bus Element1/1
  Multiply/1 -> Relational Operator/2
  Relational Operator/1 -> AKState1/1
  Logical Operator/1 -> Logical Operator2/1
  AKState1/1 -> Data Type Conversion4/1, Unit Delay/1, Data Type Conversion3/1  "KContactor"
  AKState1/2 -> Terminator1/1
  Data Type Conversion/1 -> AKState/1
  Multiply1/1 -> Exp/1
  Product3/1 -> Out Bus Element2/1
  Data Type Conversion3/1 -> TMPower/1
  Data Type Conversion4/1 -> [K], Out Bus Element/1
  In Bus Element/1 -> Switch/2
  Link_OverVoltage/1 -> Switch/1
  In Bus Element1/1 -> Switch1/2
  Switch1/1 -> Switch/3
  Link_NominalVoltage/1 -> Switch1/3
  Link_UnderVoltage/1 -> Switch1/1
  Logical Operator1/1 -> AND/2
  ContactorFault/1 -> Logical Operator2/2, Logical Operator1/1
  Logical Operator2/1 -> AND1/1
  [AK] -> Logical Operator3/1
  [K] -> Logical Operator3/2
  Logical Operator3/1 -> Data Type Conversion5/1
  Data Type Conversion5/1 -> Product3/1
  In Bus Element2/1 -> Logical Operator4/1
  In Bus Element3/1 -> Logical Operator5/1
  Logical Operator4/1 -> AND/1
  AND/1 -> AKState/2
  AND1/1 -> AKState1/2
  Logical Operator5/1 -> AND1/2
  AND2/1 -> Data Type Conversion/1
  Logical Operator6/1 -> AND2/2
  Unit Delay/1 -> Logical Operator7/2, Logical Operator1/2, Logical Operator6/1
  RC_K/1 -> Switch2/1
  Logical Operator7/1 -> Switch2/2
  RC_AK/1 -> Switch2/3
  Switch2/1 -> Product/2

== system TractionSystem/Traction (Per Vehicle)/MotorVehicle/VehicleTractionConvertersSystem/BogieTractionConverterSystem (Per Bogie) ==
  BogieTractionConverterControlIn : Inport  Partition=on  PartitionDimension=1  PartitionWidth=1  PartitionOffset=0
  MotorIn : Inport  Port=2
  BogieDynamics : Inport  Port=3  Partition=on  PartitionDimension=1  PartitionWidth=1  PartitionOffset=0
  TractionEffortVariationOverride : Inport  Port=4
  BrakingEffortVariationOverride : Inport  Port=5
  Orientation : Inport  Port=6
  TCMS : Inport  Port=7
  Bus Creator : BusCreator  Inputs=9  OutDataTypeStr=Bus: BD_TractionSystem_Int_BogieOutputs  NonVirtualBus=on
  Bus Creator1 : BusCreator  Inputs=3  OutDataTypeStr=Bus: BD_TractionSystem_Int_Vehicle_Dynamics  NonVirtualBus=on
  Bus Selector : BusSelector  OutputSignals=TractionDemandPct,DynamicBrakeTorqueDemand,Powering,Braking,Forward,Reverse,TractionTorqueAvailable,DynamicBrakeAvailable,MotorNotAvailable
  Bus Selector1 : BusSelector  OutputSignals=PowerAvailable
  Bus Selector2 : BusSelector  OutputSignals=WheelSpeed
  Data Type Conversion : DataTypeConversion
  ForEachBogie : ForEach  DisableCoverage=on
  TractionConverterSystem : Subsystem
  BogieForcesPerAxle : Outport  ConcatenationDimension=1  VectorParamsAs1DForOutWhenUnconnected=off
  BogieOutputs : Outport  Port=2  ConcatenationDimension=1  VectorParamsAs1DForOutWhenUnconnected=off
  wires:
  Bus Selector/4 -> TractionConverterSystem/4(Brake)  "<Braking>"
  Bus Selector/8 -> TractionConverterSystem/8(DynamicBrakingAvailable)  "<DynamicBrakeAvailable>"
  Bus Selector/3 -> TractionConverterSystem/3(Motor)  "<Powering>"
  TractionConverterSystem/8(BogieTractivePower) -> Bus Creator/5  "BogieTractivePower"
  Bus Selector/1 -> TractionConverterSystem/1(TractionDemandPct)  "<TractionDemandPct>"
  Orientation/1 -> TractionConverterSystem/14(VehicleOrientation)
  BogieDynamics/1 -> Bus Selector2/1
  Bus Selector/6 -> TractionConverterSystem/6(Reverse)  "<Reverse>"
  BogieTractionConverterControlIn/1 -> Bus Selector/1
  Bus Selector/7 -> TractionConverterSystem/7(AvailableTorque)  "<TractionTorqueAvailable>"
  Bus Selector/2 -> TractionConverterSystem/2(DynamicBrakeTorqueDemand)  "<DynamicBrakeTorqueDemand>"
  Bus Selector/9 -> TractionConverterSystem/9(MotorFailure)  "<MotorNotAvailable>"
  Bus Selector1/1 -> Data Type Conversion/1  "<PowerAvailable>"
  TractionConverterSystem/5(BogieDynamicBrakingEffort) -> Bus Creator/2  "BogieDynamicBrakingEffort"
  TractionConverterSystem/1(BogieTractiveBrakingEffortPerAxle) -> Bus Creator1/1  "AxleTractionBrakingForce"
  TractionConverterSystem/12(MotorSpeeds) -> Bus Creator/9  "BogieMotorSpeeds"
  Bus Selector/5 -> TractionConverterSystem/5(Forward)  "<Forward>"
  Bus Selector2/1 -> TractionConverterSystem/11(WheelSpeed)  "<WheelSpeed>"
  BrakingEffortVariationOverride/1 -> TractionConverterSystem/13(BrakingEffortVariationOverride)
  TractionEffortVariationOverride/1 -> TractionConverterSystem/12(TractiveEffortVariationOverride)
  TractionConverterSystem/6(BogieMaxTractionEffortPossible) -> Bus Creator/3  "BogieMaxTractionEffortPossible"
  TractionConverterSystem/9(BogieDynamicBrakingPower) -> Bus Creator/6  "BogieDynamicBrakingPower"
  TractionConverterSystem/4(BogieTractiveEffort) -> Bus Creator/1  "BogieTractiveEffort"
  TractionConverterSystem/7(BogieMaxBrakingEffortPossible) -> Bus Creator/4  "BogieMaxBrakingEffortPossible"
  Bus Creator/1 -> BogieOutputs/1
  TractionConverterSystem/10(BogieMaxTractionPowerPossible) -> Bus Creator/7  "BogieMaxTractionPowerPossible"
  TractionConverterSystem/11(BogieMaxBrakingPowerPossible) -> Bus Creator/8  "BogieMaxBrakingPowerPossible"
  MotorIn/1 -> Bus Selector1/1
  Data Type Conversion/1 -> TractionConverterSystem/10(AvailablePower)
  TractionConverterSystem/2(BogieTractiveEffortPerAxle) -> Bus Creator1/2  "AxleTractionForce"
  TractionConverterSystem/3(BogieBrakingEffortPerAxle) -> Bus Creator1/3  "AxleBrakingForce"
  Bus Creator1/1 -> BogieForcesPerAxle/1
  TCMS/1 -> TractionConverterSystem/15(TCMS)

== system TractionSystem/Traction (Per Vehicle)/MotorVehicle/OutputAdapter/AudioOutputsRepack/ForEachBogie ==
  BogieTraction : Inport  Partition=on  PartitionDimension=1  PartitionWidth=1  PartitionOffset=0
  BogieDynamics : Inport  Port=2  Partition=on  PartitionDimension=1  PartitionWidth=1  PartitionOffset=0
  Abs : Abs
  Bus Selector : BusSelector  OutputSignals=WheelSpeed
  Bus Selector1 : BusSelector  OutputSignals=AxleTractionBrakingForce
  For Each : ForEach  DisableCoverage=on
  IfWheelSlipping : MinMax  Function=max
  Product : Product
  Sum of Elements : Sum  Inputs=+
  BogieTractionBrakingPower : Outport  ConcatenationDimension=1
  BogieWheelSpeed : Outport  Port=2  ConcatenationDimension=1
  wires:
  BogieDynamics/1 -> Bus Selector/1
  Bus Selector/1 -> Abs/1, IfWheelSlipping/1  "<WheelSpeed>"
  BogieTraction/1 -> Bus Selector1/1
  Bus Selector1/1 -> Product/1  "<AxleTractionBrakingForce>"
  Sum of Elements/1 -> BogieTractionBrakingPower/1
  IfWheelSlipping/1 -> BogieWheelSpeed/1
  Abs/1 -> Product/2
  Product/1 -> Sum of Elements/1

== system TractionSystem/Traction (Per Vehicle)/MotorVehicle/OutputAdapter/DynamicsOutputsRepack/For Each Subsystem ==
  In1 : Inport  Partition=on  PartitionDimension=1  PartitionWidth=1  PartitionOffset=0
  Bus Selector : BusSelector  OutputSignals=AxleTractionBrakingForce,AxleTractionForce,AxleBrakingForce
  For Each : ForEach  DisableCoverage=on
  TractionBrakingForce : Outport  ConcatenationDimension=1
  TractionForce : Outport  Port=2  ConcatenationDimension=1
  BrakingForce : Outport  Port=3  ConcatenationDimension=1
  wires:
  In1/1 -> Bus Selector/1
  Bus Selector/1 -> TractionBrakingForce/1  "<AxleTractionBrakingForce>"
  Bus Selector/2 -> TractionForce/1  "<AxleTractionForce>"
  Bus Selector/3 -> BrakingForce/1  "<AxleBrakingForce>"

== system TractionSystem/Traction (Per Vehicle)/MotorVehicle/VehicleTractionControlUnit/OutputAdapter/BCUOutputsRepack ==
  In1 : Inport
  Bus Assignment2 : BusAssignment  AssignedSignals=Bogie
  Constant2 : Constant  Value=0  OutDataTypeStr=Bus: BD_TractionSystem_Out_Vehicle_BCU
  ToBCU : Outport
  wires:
  Bus Assignment2/1 -> ToBCU/1
  In1/1 -> Bus Assignment2/2
  Constant2/1 -> Bus Assignment2/1

== system TractionSystem/Traction (Per Vehicle)/MotorVehicle/VehicleTractionControlUnit/OutputAdapter/ElectricalOutputsRepack ==
  In2 : Inport
  In1 : Inport  Port=2
  Bus Assignment2 : BusAssignment  AssignedSignals=Bogie,TractionContactorStatus
  Constant2 : Constant  Value=0  OutDataTypeStr=Bus: BD_TractionSystem_Out_Vehicle_ElectricalSystem
  ToElectrical : Outport
  wires:
  Constant2/1 -> Bus Assignment2/1
  In1/1 -> Bus Assignment2/2
  Bus Assignment2/1 -> ToElectrical/1
  In2/1 -> Bus Assignment2/3

== system TractionSystem/Traction (Per Vehicle)/MotorVehicle/VehicleTractionControlUnit/OutputAdapter/TCMSOutputsRepack ==
  In1 : Inport
  In2 : Inport  Port=2
  In3 : Inport  Port=3
  Bus Assignment1 : BusAssignment  AssignedSignals=Bogie,Trafo_TCU,VehicleDerailed,VehicleBogieDerailed
  Bus Selector : BusSelector  OutputSignals=DerailmentDetectedRightSide,BogieDerailed
  Constant4 : Constant  Value=0  OutDataTypeStr=Bus: BD_TractionSystem_Out_Vehicle_TCMS
  ToTCMS : Outport
  wires:
  Bus Assignment1/1 -> ToTCMS/1  "ToTCMS"
  In1/1 -> Bus Assignment1/2
  Constant4/1 -> Bus Assignment1/1
  In2/1 -> Bus Assignment1/3
  Bus Selector/1 -> Bus Assignment1/4  "<DerailmentDetectedRightSide>"
  Bus Selector/2 -> Bus Assignment1/5  "<BogieDerailed>"
  In3/1 -> Bus Selector/1

== system TractionSystem/Traction (Per Vehicle)/MotorVehicle/VehicleTractionControlUnit/TractionControl (Per Bogie)/Subsystem ==
  Velocity : Inport
  <BECU1FailureAllSpeedSensors> : Inport  Port=2
  AND : Logic  AllPortsSameDT=off  OutDataTypeStr=boolean
  Abs : Abs
  Compare To Constant : simulink/Logic and Bit Operations/Compare To Constant  relop=>  const=0.1  OutDataTypeStr=boolean
  Constant : Constant  Value=0
  Data Type Conversion : DataTypeConversion
  Detect Decrease : simulink/Logic and Bit Operations/Detect Decrease  vinit=0.0  OutDataTypeStr=boolean
  Mux : Mux  Inputs=2
  SR Latch - Reset Priority : LatchesLib/SR Latch - Reset Priority  initial_condition=0
      settings: SourceProductName=Latches
  Switch : Switch  Criteria=u2 > Threshold
  VelocityWithSensor : Outport
  wires:
  Compare To Constant/1 -> AND/1
  Velocity/1 -> Abs/1, Switch/3
  AND/1 -> SR Latch - Reset Priority/1  "SpeedSensorFault"
  Switch/1 -> Mux/2  "Velocity"
  Constant/1 -> Switch/1
  Mux/1 -> VelocityWithSensor/1
  <BECU1FailureAllSpeedSensors>/1 -> Switch/2, Detect Decrease/1, AND/2
  Data Type Conversion/1 -> Mux/1
  Abs/1 -> Compare To Constant/1
  SR Latch - Reset Priority/1 -> Data Type Conversion/1
  Detect Decrease/1 -> SR Latch - Reset Priority/2

== system TractionSystem/Traction (Per Vehicle)/MotorVehicle/VehicleTractionControlUnit/TractionControl (Per Bogie)/TCUOFFLogic ==
  Action Port : ActionPort  ActionPortLabel=else
  Constant1 : Constant  Value=0  OutDataTypeStr=Bus: BD_TractionSystem_Out_Vehicle_TCMS_Bogie
  Constant2 : Constant  Value=0  OutDataTypeStr=Bus: BD_TractionSystem_Out_Vehicle_BCU_Bogie
  Constant3 : Constant  Value=0  OutDataTypeStr=Bus: BD_TractionSystem_Int_BogieControl
  Constant4 : Constant  Value=0  OutDataTypeStr=Bus: BD_TractionSystem_Out_Vehicle_ElectricalSystem_Bogie
  TractionConverterControlOut : Outport
  TCUtoElectricalOut : Outport  Port=2
  TCUtoTCMSOut : Outport  Port=3
  TCUToBCUOut : Outport  Port=4
  wires:
  Constant4/1 -> TCUtoElectricalOut/1
  Constant1/1 -> TCUtoTCMSOut/1
  Constant2/1 -> TCUToBCUOut/1
  Constant3/1 -> TractionConverterControlOut/1

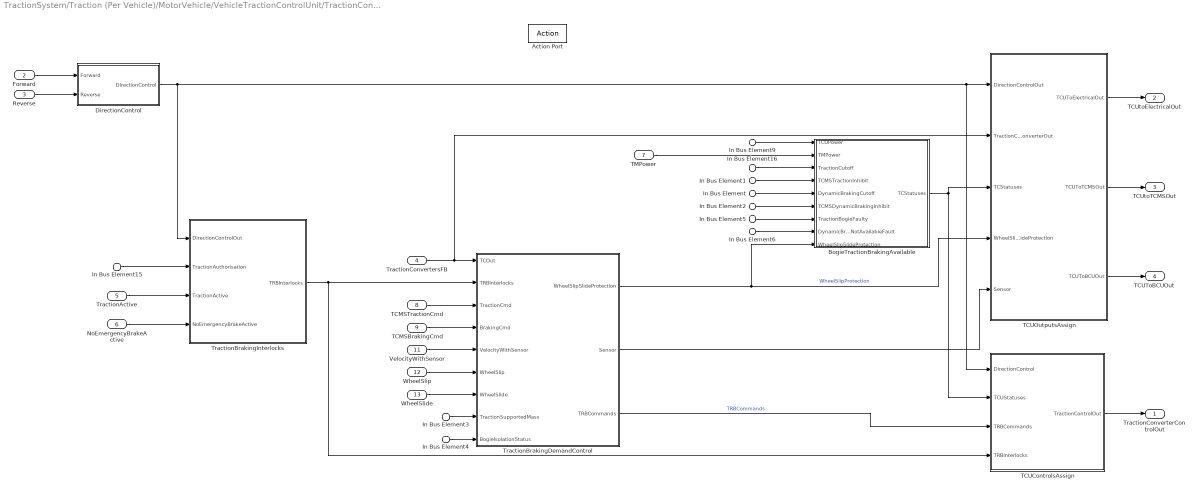
== system TractionSystem/Traction (Per Vehicle)/MotorVehicle/VehicleTractionControlUnit/TractionControl (Per Bogie)/TCUONLogic ==
  In Bus Element9 : Inport  PortName=BogieElectrical  Element=TCUPower
  In Bus Element15 : Inport  PortName=BogieElectrical  Element=TractionAuthorisation
  In Bus Element16 : Inport  PortName=BogieElectrical  Element=TractionCutoff
  In Bus Element : Inport  PortName=BogieElectrical  Element=DynamicBrakingCutoff
  Forward : Inport  Port=2
  Reverse : Inport  Port=3
  TractionConvertersFB : Inport  Port=4
  TractionActive : Inport  Port=5
  NoEmergencyBrakeActive : Inport  Port=6
  TMPower : Inport  Port=7
  TCMSTractionCmd : Inport  Port=8
  TCMSBrakingCmd : Inport  Port=9
  In Bus Element1 : Inport  Port=10  PortName=TCMSBogie  Element=TCMSTractionInhibit
  In Bus Element2 : Inport  Port=10  PortName=TCMSBogie  Element=TCMSDynamicBrakingInhibit
  In Bus Element3 : Inport  Port=10  PortName=TCMSBogie  Element=BogieSupportedMass
  In Bus Element4 : Inport  Port=10  PortName=TCMSBogie  Element=BogieIsolationStatus
  VelocityWithSensor : Inport  Port=11
  WheelSlip : Inport  Port=12
  WheelSlide : Inport  Port=13
  In Bus Element5 : Inport  Port=14  PortName=BogieFaults  Element=TractionBogieFaulty
  In Bus Element6 : Inport  Port=14  PortName=BogieFaults  Element=DynamicBrakeNotAvailable
  Action Port : ActionPort  ActionPortLabel=if(u1 > 0)
  BogieTractionBrakingAvailable : Subsystem
  DirectionControl : Subsystem
  TCUControlsAssign : Subsystem
  TCUOutputsAssign : Subsystem
  TractionBrakingDemandControl : Subsystem  mask(Traction and Braking Demands Control){NumberOfMotors=Prm_TractionSystem.DesignBogieMotorCount, GearRatio=Prm_TractionSystem.DesignGearingRatio, WheelDiam=Prm_TractionSystem.DesignWheelDiameter, BrakeFadeSpeed=Prm_TractionSystem.BrakeFadeRampDownSpeeds(2), BrakeFadeTime=0.4, WheelSlipProtectionEnable=Prm_TractionSystem.WheelSlipProtectionEnable, WheelSlideProtectionEnable=Prm_TractionSystem.WheelSlideProtectionEnable, JerkLimit=Prm_TractionSystem.JerkLimit, MaxSlipTime=Prm_TractionSystem.MaxContinuousSlipBeforeTractionCutout, MaxSlideTime=Prm_TractionSystem.MaxContinuousSlideBeforeBrakeCutout}
      mask prompts: NumberOfMotors "Number of Motors per bogie [-]"; GearRatio "Gear Ratio [-]"; WheelDiam "Wheel Diameter [m]"; BrakeFadeSpeed "ED Brake Fade Start Speed [m/s]"; BrakeFadeTime "ED Brake Fade Heads Up Timing [s]"; WheelSlipProtectionEnable "Enable Wheel Slip Protection"; WheelSlideProtectionEnable "Enable Wheel Slide Protection"; JerkLimit "Jerk Limit [m/s3]"; MaxSlipTime "Maximum Continuous Slip Duration before Traction Cutout [s]"; MaxSlideTime "Maximum Continuous Slide Duration before Brake Cutout [s]"
      mask help:
      | ED Brake Fade
      | The "Heads-Up Time" describes the delay between the moment the TCU notifies the BCU that the brakes are going to fade (so that it prepares for a pneumatic application) and the moment dynamic brake actually starts to fade.
      mask DialogControl Container7 Prompt: General
      mask DialogControl Container8 Prompt: Brake Fade
      mask DialogControl Container12 Prompt: Wheel Slip/Slide Protection
  TractionBrakingInterlocks : Subsystem  mask{EBdeactivateED=Prm_TractionSystem.EmergencyBrakeDeactivatesDynamicBrake}
      mask prompts: EBdeactivateED "Emergency Brake Deactivates Braking Interlock"
  TractionConverterControlOut : Outport
  TCUtoElectricalOut : Outport  Port=2
  TCUtoTCMSOut : Outport  Port=3
  TCUToBCUOut : Outport  Port=4
  wires:
  TCUOutputsAssign/1(TCUToElectricalOut) -> TCUtoElectricalOut/1
  TCUControlsAssign/1(TractionControlOut) -> TractionConverterControlOut/1
  DirectionControl/1(DirectionControl) -> TractionBrakingInterlocks/1(DirectionControlOut), TCUControlsAssign/1(DirectionControl), TCUOutputsAssign/1(DirectionControlOut)
  BogieTractionBrakingAvailable/1(TCStatuses) -> TCUControlsAssign/2(TCUStatuses), TCUOutputsAssign/3(TCStatuses)
  Forward/1 -> DirectionControl/1(Forward)
  Reverse/1 -> DirectionControl/2(Reverse)
  In Bus Element9/1 -> BogieTractionBrakingAvailable/1(TCUPower)
  In Bus Element15/1 -> TractionBrakingInterlocks/2(TractionAuthorisation)
  In Bus Element16/1 -> BogieTractionBrakingAvailable/3(TractionCutoff)
  TractionActive/1 -> TractionBrakingInterlocks/3(TractionActive)
  NoEmergencyBrakeActive/1 -> TractionBrakingInterlocks/4(NoEmergencyBrakeActive)
  TCUOutputsAssign/2(TCUToTCMSOut) -> TCUtoTCMSOut/1
  TCUOutputsAssign/3(TCUToBCUOut) -> TCUToBCUOut/1
  In Bus Element1/1 -> BogieTractionBrakingAvailable/4(TCMSTractionInhibit)
  In Bus Element/1 -> BogieTractionBrakingAvailable/5(DynamicBrakingCutoff)
  In Bus Element2/1 -> BogieTractionBrakingAvailable/6(TCMSDynamicBrakingInhibit)
  In Bus Element3/1 -> TractionBrakingDemandControl/8(TractionSupportedMass)
  WheelSlide/1 -> TractionBrakingDemandControl/7(WheelSlide)
  WheelSlip/1 -> TractionBrakingDemandControl/6(WheelSlip)
  VelocityWithSensor/1 -> TractionBrakingDemandControl/5(VelocityWithSensor)
  TCMSBrakingCmd/1 -> TractionBrakingDemandControl/4(BrakingCmd)
  TractionBrakingInterlocks/1(TRBInterlocks) -> TCUControlsAssign/4(TRBInterlocks), TractionBrakingDemandControl/2(TRBInterlocks)
  TractionBrakingDemandControl/1(WheelSlipSlideProtection) -> BogieTractionBrakingAvailable/9(WheelSlipSlideProtection), TCUOutputsAssign/4(WheelSlipSlideProtection)  "WheelSlipProtection"
  TractionBrakingDemandControl/3(TRBCommands) -> TCUControlsAssign/3(TRBCommands)  "TRBCommands"
  TCMSTractionCmd/1 -> TractionBrakingDemandControl/3(TractionCmd)
  TractionConvertersFB/1 -> TractionBrakingDemandControl/1(TCOut), TCUOutputsAssign/2(TractionConverterOut)
  In Bus Element5/1 -> BogieTractionBrakingAvailable/7(TractionBogieFaulty)
  In Bus Element6/1 -> BogieTractionBrakingAvailable/8(DynamicBrakeNotAvailableFault)
  TMPower/1 -> BogieTractionBrakingAvailable/2(TMPower)
  TractionBrakingDemandControl/2(Sensor) -> TCUOutputsAssign/5(Sensor)
  In Bus Element4/1 -> TractionBrakingDemandControl/9(BogieIsolationStatus)
